simulink model "Test3"  (R2025b)
settings: Solver=VariableStepAuto  StartTime=0.0  StopTime=10.0  RelTol=1e-3
libraries: simulink x7
settings Model: Creator=henni  LastModifiedBy=henni

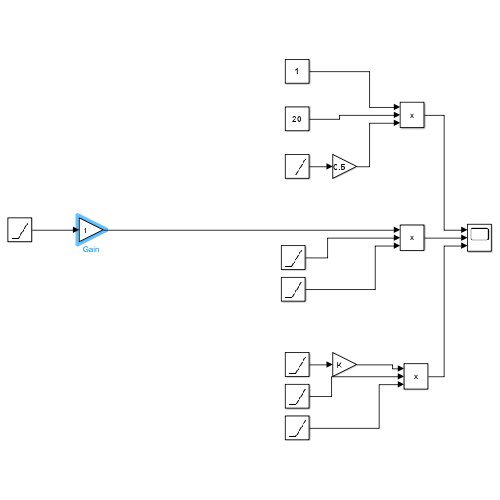
[thumbnail: Simulink's stored preview of the top-level diagram]
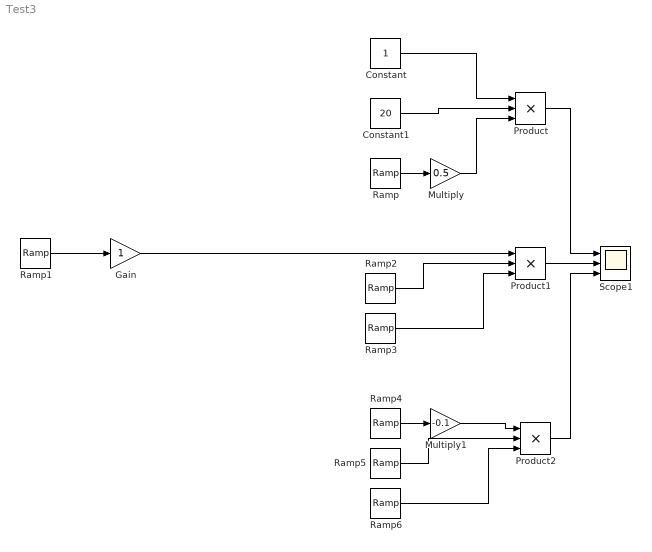
== system Test3 ==
  Constant : Constant
  Constant1 : Constant  Value=20
  Gain : Gain
  Multiply : Gain  Gain=0.5
  Multiply1 : Gain  Gain=-0.1
  Product : Product  Inputs=3
  Product1 : Product  Inputs=3
  Product2 : Product  Inputs=3
  Ramp : simulink/Sources/Ramp  slope=1  start=0  InitialOutput=0
  Ramp1 : simulink/Sources/Ramp  slope=5  start=0  InitialOutput=0
  Ramp2 : simulink/Sources/Ramp  slope=2  start=0  InitialOutput=0
  Ramp3 : simulink/Sources/Ramp  slope=-6  start=0  InitialOutput=5
  Ramp4 : simulink/Sources/Ramp  slope=5  start=0  InitialOutput=0
  Ramp5 : simulink/Sources/Ramp  slope=2  start=0  InitialOutput=0
  Ramp6 : simulink/Sources/Ramp  slope=-6  start=0  InitialOutput=5
  Scope1 : Scope  NumInputPorts=3
      settings: ActiveDisplayYMinimum=-61875.63  ActiveDisplayYMaximum=6880.6699999999983
  wires:
  Ramp/1 -> Multiply/1
  Constant1/1 -> Product/2
  Constant/1 -> Product/1
  Product/1 -> Scope1/1
  Ramp1/1 -> Gain/1
  Ramp2/1 -> Product1/2
  Ramp3/1 -> Product1/3
  Product1/1 -> Scope1/2
  Product2/1 -> Scope1/3
  Ramp5/1 -> Product2/2
  Ramp6/1 -> Product2/3
  Ramp4/1 -> Multiply1/1
  Multiply/1 -> Product/3
  Multiply1/1 -> Product2/1
  Gain/1 -> Product1/1
